simulink model "Static_Control"  (R2015b)
settings: Solver=VariableStepAuto  StartTime=0  StopTime=26  RelTol=1e-3
values from neighbouring files (symbols this model uses):
  Beta0 = pi    (= 3.14159265359)    [init.m]
  d = 0.15    [init.m]
  Kp1 = Kp    (= 4)    [init.m]
  Kp2 = Kp    (= 4)    [init.m]
  L = 0.13    [init.m]
  r = 0.1    [init.m]
  R = 2    [init.m]
  Theta0 = pi    (= 3.14159265359)    [init.m]
  wd = 0.5    [init.m]
  X0 = 2.3    [init.m]
  Y0 = 0    [init.m]
undefined symbols (not defined in the file): alpha
libraries: simulink x2
settings Model: Creator=GANESH  LastModifiedBy=GANESH

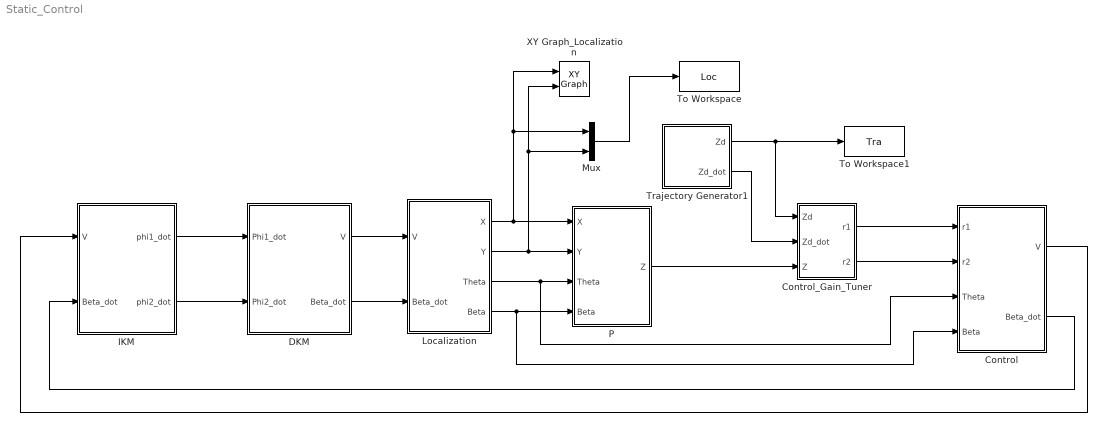
== system Static_Control ==
  Control : Subsystem  mask{r=r, L=L, d=d}
      mask prompts: r "Radius of the wheels"; L "Half of WheelBase"; d "Distance of Point P"
  Control_Gain_Tuner : Subsystem
  DKM : Subsystem  mask{r=r}
      mask prompts: r "Radius of the wheels"
  IKM : Subsystem  mask{r=(1+alpha)*r}
      mask prompts: r "Radius of the Wheels"
  Localization : Subsystem  mask{L=L}
      mask prompts: L "Half of WheelBase"
  Mux : Mux  Inputs=2
  P : Subsystem  mask{d=d, L=L}
      mask prompts: d "Distance of Point P"; L "Half of WheelBase"
  To Workspace : ToWorkspace  VariableName=Loc  SaveFormat=Timeseries  SampleTime=-1
  To Workspace1 : ToWorkspace  VariableName=Tra  SaveFormat=Timeseries  SampleTime=-1
  Trajectory Generator1 : Subsystem
  XY Graph_Localization : simulink/Sinks/XY Graph  xmin=-5  xmax=5  ymin=-5  ymax=5  st=-1
  wires:
  IKM/2(phi2_dot) -> DKM/2(Phi2_dot)
  P/1(Z) -> Control_Gain_Tuner/3(Z)
  Trajectory Generator1/1(Zd) -> Control_Gain_Tuner/1(Zd), To Workspace1/1
  Trajectory Generator1/2(Zd_dot) -> Control_Gain_Tuner/2(Zd_dot)
  IKM/1(phi1_dot) -> DKM/1(Phi1_dot)
  DKM/1(V) -> Localization/1(V)
  DKM/2(Beta_dot) -> Localization/2(Beta_dot)
  Control_Gain_Tuner/1(r1) -> Control/1(r1)
  Control_Gain_Tuner/2(r2) -> Control/2(r2)
  Control/1(V) -> IKM/1(V)
  Control/2(Beta_dot) -> IKM/2(Beta_dot)
  Localization/1(X) -> XY Graph_Localization/1, Mux/1, P/1(X)
  Localization/2(Y) -> Mux/2, XY Graph_Localization/2, P/2(Y)
  Localization/3(Theta) -> P/3(Theta), Control/3(Theta)
  Localization/4(Beta) -> Control/4(Beta), P/4(Beta)
  Mux/1 -> To Workspace/1

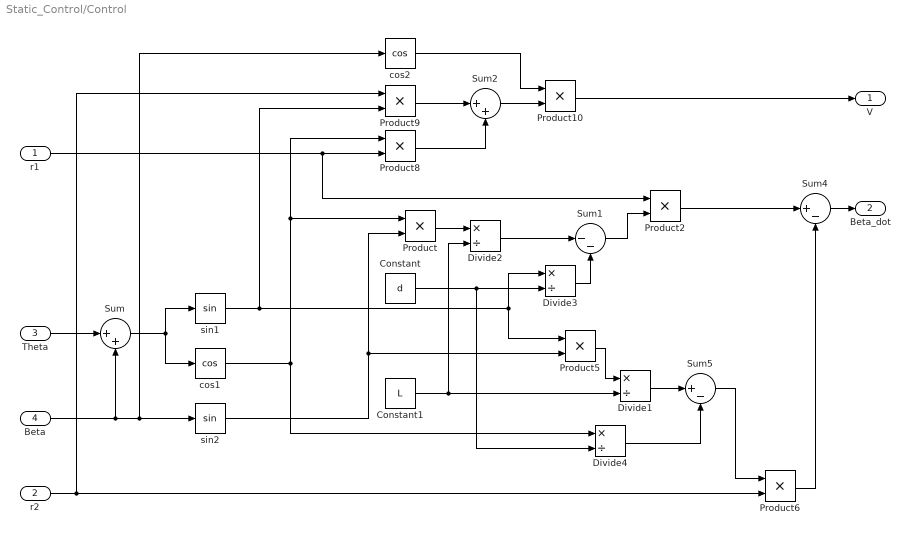
== system Static_Control/Control ==
  r1 : Inport
  r2 : Inport  Port=2
  Theta : Inport  Port=3
  Beta : Inport  Port=4
  Constant : Constant  Value=d
  Constant1 : Constant  Value=L
  Divide{1..4} (4 alike) : Product  Inputs=*/
  Product{,2,5..6,8..10} (7 alike) : Product
  Sum : Sum  Inputs=|++
  Sum1 : Sum  Inputs=|--
  Sum2 : Sum  Inputs=|++
  Sum4 : Sum  Inputs=|+-
  Sum5 : Sum  Inputs=|+-
  cos1 : Trigonometry  Operator=cos
  cos2 : Trigonometry  Operator=cos
  sin1 : Trigonometry
  sin2 : Trigonometry
  V : Outport
  Beta_dot : Outport  Port=2
  wires:
  Theta/1 -> Sum/1
  r1/1 -> Product8/2, Product2/1
  sin1/1 -> Divide3/1, Product5/1, Product9/2
  cos1/1 -> Product8/1, Product/1, Divide4/1
  Product/1 -> Divide2/1
  Beta/1 -> Sum/2, cos2/1, sin2/1
  Divide2/1 -> Sum1/1
  Sum/1 -> sin1/1, cos1/1
  sin2/1 -> Product5/2, Product/2
  Constant1/1 -> Divide2/2, Divide1/2
  Divide3/1 -> Sum1/2
  Product2/1 -> Sum4/1
  Constant/1 -> Divide3/2, Divide4/2
  Sum5/1 -> Product6/1
  Divide1/1 -> Sum5/1
  r2/1 -> Product9/1, Product6/2
  Product5/1 -> Divide1/1
  Sum4/1 -> Beta_dot/1
  Divide4/1 -> Sum5/2
  Product6/1 -> Sum4/2
  Product9/1 -> Sum2/1
  Product8/1 -> Sum2/2
  Sum2/1 -> Product10/2
  cos2/1 -> Product10/1
  Product10/1 -> V/1
  Sum1/1 -> Product2/2

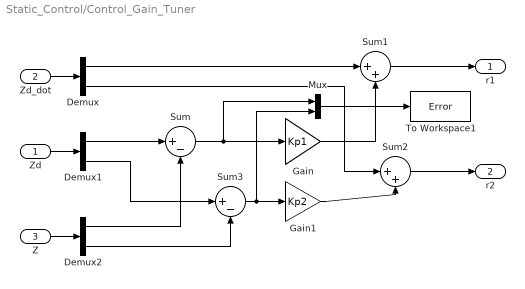
== system Static_Control/Control_Gain_Tuner ==
  Zd : Inport
  Zd_dot : Inport  Port=2
  Z : Inport  Port=3
  Demux : Demux  Outputs=2
  Demux1 : Demux  Outputs=2
  Demux2 : Demux  Outputs=2
  Gain : Gain  Gain=Kp1
  Gain1 : Gain  Gain=Kp2
  Mux : Mux  Inputs=2
  Sum : Sum  Inputs=|+-
  Sum1 : Sum  Inputs=|++
  Sum2 : Sum  Inputs=|++
  Sum3 : Sum  Inputs=|+-
  To Workspace1 : ToWorkspace  VariableName=Error  SaveFormat=Timeseries  SampleTime=-1
  r1 : Outport
  r2 : Outport  Port=2
  wires:
  Demux2/2 -> Sum3/2
  Demux1/1 -> Sum/1
  Gain/1 -> Sum1/2
  Demux2/1 -> Sum/2
  Zd_dot/1 -> Demux/1
  Gain1/1 -> Sum2/2
  Demux/1 -> Sum1/1
  Sum3/1 -> Mux/2, Gain1/1
  Demux1/2 -> Sum3/1
  Sum1/1 -> r1/1
  Zd/1 -> Demux1/1
  Sum2/1 -> r2/1
  Sum/1 -> Mux/1, Gain/1
  Z/1 -> Demux2/1
  Demux/2 -> Sum2/1
  Mux/1 -> To Workspace1/1

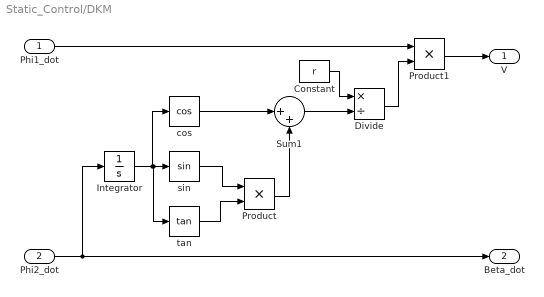
== system Static_Control/DKM ==
  Phi1_dot : Inport
  Phi2_dot : Inport  Port=2
  Constant : Constant  Value=r
  Divide : Product  Inputs=*/
  Integrator : Integrator  InitialCondition=Beta0
  Product : Product
  Product1 : Product
  Sum1 : Sum  Inputs=|++
  cos : Trigonometry  Operator=cos
  sin : Trigonometry
  tan : Trigonometry  Operator=tan
  V : Outport
  Beta_dot : Outport  Port=2
  wires:
  Divide/1 -> Product1/2
  Phi1_dot/1 -> Product1/1
  Product/1 -> Sum1/2
  Phi2_dot/1 -> Beta_dot/1, Integrator/1
  Integrator/1 -> tan/1, sin/1, cos/1
  sin/1 -> Product/1
  tan/1 -> Product/2
  Sum1/1 -> Divide/2
  Constant/1 -> Divide/1
  Product1/1 -> V/1
  cos/1 -> Sum1/1

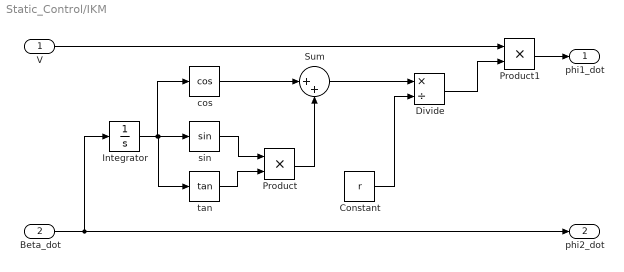
== system Static_Control/IKM ==
  V : Inport
  Beta_dot : Inport  Port=2
  Constant : Constant  Value=r
  Divide : Product  Inputs=*/
  Integrator : Integrator  InitialCondition=Beta0
  Product : Product
  Product1 : Product
  Sum : Sum  Inputs=|++
  cos : Trigonometry  Operator=cos
  sin : Trigonometry
  tan : Trigonometry  Operator=tan
  phi1_dot : Outport
  phi2_dot : Outport  Port=2
  wires:
  Constant/1 -> Divide/2
  Divide/1 -> Product1/2
  V/1 -> Product1/1
  Product/1 -> Sum/2
  Beta_dot/1 -> phi2_dot/1, Integrator/1
  Sum/1 -> Divide/1
  Integrator/1 -> tan/1, sin/1, cos/1
  sin/1 -> Product/1
  tan/1 -> Product/2
  Product1/1 -> phi1_dot/1
  cos/1 -> Sum/1

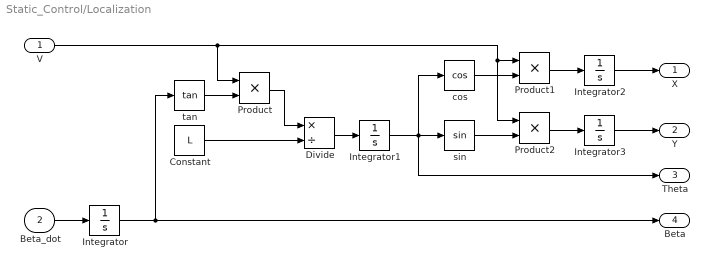
== system Static_Control/Localization ==
  V : Inport
  Beta_dot : Inport  Port=2
  Constant : Constant  Value=L
  Divide : Product  Inputs=*/
  Integrator : Integrator  InitialCondition=Beta0
  Integrator1 : Integrator  InitialCondition=Theta0
  Integrator2 : Integrator  InitialCondition=X0
  Integrator3 : Integrator  InitialCondition=Y0
  Product : Product
  Product1 : Product
  Product2 : Product
  "cos " : Trigonometry  Operator=cos
  sin : Trigonometry
  tan : Trigonometry  Operator=tan
  X : Outport
  Y : Outport  Port=2
  Theta : Outport  Port=3
  Beta : Outport  Port=4
  wires:
  Integrator1/1 -> Theta/1, "cos "/1, sin/1
  Product2/1 -> Integrator3/1
  Integrator3/1 -> Y/1
  V/1 -> Product1/1, Product2/1, Product/1
  Product/1 -> Divide/1
  Integrator/1 -> Beta/1, tan/1
  Product1/1 -> Integrator2/1
  Integrator2/1 -> X/1
  "cos "/1 -> Product1/2
  Divide/1 -> Integrator1/1
  Beta_dot/1 -> Integrator/1
  tan/1 -> Product/2
  sin/1 -> Product2/2
  Constant/1 -> Divide/2

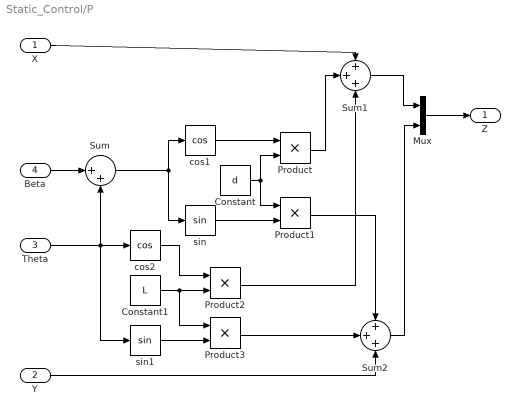
== system Static_Control/P ==
  X : Inport
  Y : Inport  Port=2
  Theta : Inport  Port=3
  Beta : Inport  Port=4
  Constant : Constant  Value=d
  Constant1 : Constant  Value=L
  Mux : Mux  Inputs=2
  Product{,1..3} (4 alike) : Product
  Sum : Sum  Inputs=|++
  Sum1 : Sum  Inputs=+++
  Sum2 : Sum  Inputs=+++
  cos1 : Trigonometry  Operator=cos
  cos2 : Trigonometry  Operator=cos
  sin : Trigonometry
  sin1 : Trigonometry
  Z : Outport
  wires:
  Theta/1 -> sin1/1, Sum/2, cos2/1
  Mux/1 -> Z/1
  Sum1/1 -> Mux/1
  cos2/1 -> Product2/1
  X/1 -> Sum1/1
  Sum/1 -> sin/1, cos1/1
  Beta/1 -> Sum/1
  Sum2/1 -> Mux/2
  sin/1 -> Product1/2
  cos1/1 -> Product/1
  Product3/1 -> Sum2/2
  Product/1 -> Sum1/2
  Constant1/1 -> Product2/2, Product3/1
  Constant/1 -> Product1/1, Product/2
  sin1/1 -> Product3/2
  Product1/1 -> Sum2/1
  Y/1 -> Sum2/3
  Product2/1 -> Sum1/3

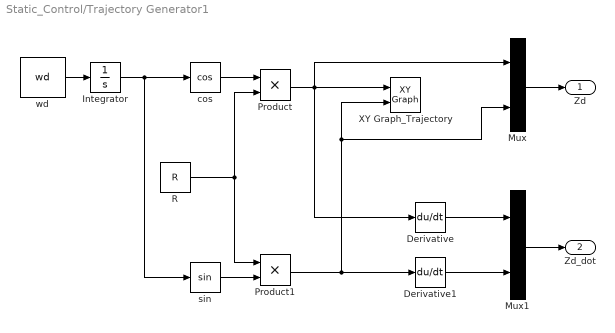
== system Static_Control/Trajectory Generator1 ==
  Derivative : Derivative
  Derivative1 : Derivative
  Integrator : Integrator
  Mux : Mux  Inputs=2
  Mux1 : Mux  Inputs=2
  Product : Product
  Product1 : Product
  R : Constant  Value=R
  XY Graph_Trajectory : simulink/Sinks/XY Graph  xmin=-5  xmax=5  ymin=-5  ymax=5  st=-1
  cos : Trigonometry  Operator=cos
  sin : Trigonometry
  wd : Constant  Value=wd
  Zd : Outport
  Zd_dot : Outport  Port=2
  wires:
  Mux/1 -> Zd/1
  R/1 -> Product1/1, Product/2
  Product1/1 -> Derivative1/1, Mux/2, XY Graph_Trajectory/2
  wd/1 -> Integrator/1
  cos/1 -> Product/1
  Integrator/1 -> cos/1, sin/1
  sin/1 -> Product1/2
  Derivative/1 -> Mux1/1
  Derivative1/1 -> Mux1/2
  Mux1/1 -> Zd_dot/1
  Product/1 -> Mux/1, XY Graph_Trajectory/1, Derivative/1
